simulink model "pendulum_test_model"  (R2024b)
settings: Solver=ode3  StartTime=0.0  StopTime=t(end)  RelTol=1e-3
values from neighbouring files (symbols this model uses):
  fi_dc0 = 0    [currwork.mat]    (also in pendulum_friction_coefficient_identification.m)
  g = 9.81    [currwork.mat]    (also in pendulum_friction_coefficient_identification.m)
  J_pend = 0.026668518142893    (= 0.0266685181429)    [pendulum_friction_coefficient_identification.m]
  kr = 0.026    [currwork.mat]
  kt = 0.026    [currwork.mat]
  omega_dc0 = 0    [currwork.mat]    (also in pendulum_friction_coefficient_identification.m)
  omega_pend0 = 0    [currwork.mat]    (also in pendulum_friction_coefficient_identification.m)
  R = 2.4    [currwork.mat]
  U = 0.012144    [currwork.mat]    (also in pendulum_friction_coefficient_identification.m)
  uc_dc = 0.0016    [currwork.mat]
  uc_pend = 0.00434561903982    [currwork.mat]    (also in pendulum_friction_coefficient_identification.m)
  uv_dc = 5.3017e-06    [currwork.mat]
  uv_pend = 0.000184765206116    [currwork.mat]    (also in pendulum_friction_coefficient_identification.m)
undefined symbols (not defined in the file or in its folder): J_rotor, sigbuilder_block
settings Model: Creator=Student  LastModifiedBy=Paweł Wiktor
settings SolverCC: AlgebraicLoopSolver=TrustRegion
settings DataIOCC: ReturnWorkspaceOutputs=off
settings DebuggingCC: UnconnectedInputMsg=warning  UnconnectedOutputMsg=warning  UnconnectedLineMsg=warning  ArithmeticOperatorsInVariantConditions=warning
settings ModelReferenceCC: EnableRefExpFcnMdlSchedulingChecks=on
settings SFSimCC: CustomCodeUndefinedFunction=UseInterfaceOnly
settings RTWCC: GPUComputeCapability=3.5

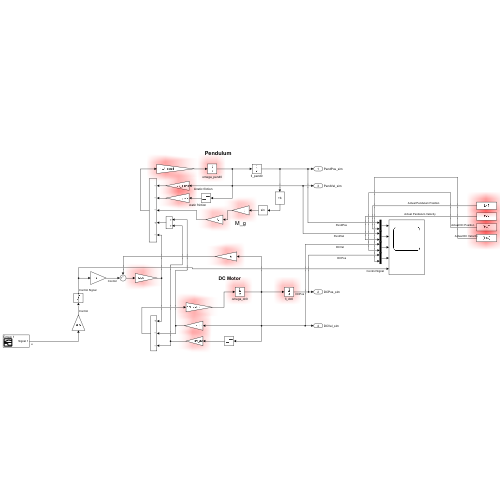
[thumbnail: Simulink's stored preview of the top-level diagram]
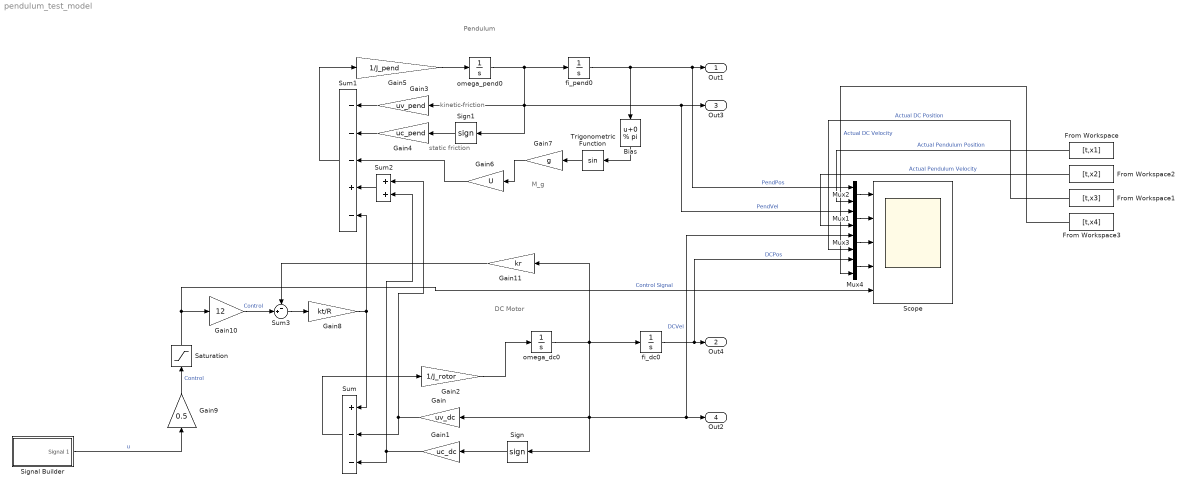
== system pendulum_test_model ==
  note: DC Motor
  note: Pendulum
  note: kinetic friction
  note: static friction
  note: M_g
  Bias : Bias  Bias=0 % pi  SaturateOnIntegerOverflow=off
  From Workspace : FromWorkspace  VariableName=[t,x1]
  From Workspace1 : FromWorkspace  VariableName=[t,x3]
  From Workspace2 : FromWorkspace  VariableName=[t,x2]
  From Workspace3 : FromWorkspace  VariableName=[t,x4]
  Gain : Gain  Gain=uv_dc
  Gain1 : Gain  Gain=uc_dc
  Gain10 : Gain  Gain=12
  Gain11 : Gain  Gain=kr
  Gain2 : Gain  Gain=1/J_rotor
  Gain3 : Gain  Gain=uv_pend
  Gain4 : Gain  Gain=uc_pend
  Gain5 : Gain  Gain=1/J_pend
  Gain6 : Gain  Gain=U
  Gain7 : Gain  Gain=g
  Gain8 : Gain  Gain=kt/R
  Gain9 : Gain  Gain=0.5
  Mux{1..4} (4 alike) : Mux  Inputs=2
  Saturation : Saturate  UpperLimit=1  LowerLimit=-1
  Scope : Scope  NumInputPorts=5
  Sign : Signum  ZeroCross=off
  Sign1 : Signum  ZeroCross=off
  Signal Builder : Subsystem  Tag=STV Subsys  LoadFcn=sigbuilder_block('load');  StartFcn=sigbuilder_block('start');  StopFcn=sigbuilder_block('stop');  ClipboardFcn=sigbuilder_block('clipboard');  mask(Sigbuilder block){tuvar=[0:10]}
      mask help: Simulink:masks:SigbuilderBlock_MD
      mask init:
      | if ~strcmp(get_param(bdroot(gcbh),'SimulationStatus'),'stopped') tuvar = sigbuilder_block('maskInit'); end
      settings: CopyFcn=sigbuilder_block('copy');  DeleteFcn=sigbuilder_block('delete');  ModelCloseFcn=sigbuilder_block('modelClose');  PreSaveFcn=sigbuilder_block('preSave');  PauseFcn=sigbuilder_block('pause');  ContinueFcn=sigbuilder_block('continue');  NameChangeFcn=sigbuilder_block('namechange');  OpenFcn=sigbuilder_block('open',[0 22.5 1440 729.75 ]);  CloseFcn=sigbuilder_block('close');
      mask Display: plot(0, 0, 100, 100,[2, 2, 32, 32, 2], [68, 8, 8, 68, 68],[32, 2], [38, 38], [32, 19, 2],[53, 60, 44], [32, 17, 17, 2],[16, 16, 31, 31]);txt = getActiveGroup(gcbh);text(2, 100, txt,'verticalAlignment', 'top');
  Sum : Sum  Inputs=+--
  Sum1 : Sum  Inputs=---+-
  Sum2 : Sum
  Sum3 : Sum  Inputs=-+|
  Trigonometric Function : Trigonometry
  fi_dc0 : Integrator  InitialCondition=fi_dc0
  fi_pend0 : Integrator  InitialCondition=0.5
  omega_dc0 : Integrator  InitialCondition=omega_dc0
  omega_pend0 : Integrator  InitialCondition=omega_pend0
  Out1 : Outport  SignalName=PendPos_sim  VectorParamsAs1DForOutWhenUnconnected=off
  Out4 : Outport  Port=2  SignalName=DCPos_sim  VectorParamsAs1DForOutWhenUnconnected=off
  Out3 : Outport  Port=3  SignalName=PendVel_sim  VectorParamsAs1DForOutWhenUnconnected=off
  Out2 : Outport  Port=4  SignalName=DCVel_sim  VectorParamsAs1DForOutWhenUnconnected=off
  wires:
  omega_dc0/1 -> Gain11/1, fi_dc0/1, Mux3/1, Out2/1, Sign/1, Gain/1  "DCVel"
  Gain2/1 -> omega_dc0/1
  Sum/1 -> Gain2/1
  Sign/1 -> Gain1/1
  Gain6/1 -> Sum1/3
  Gain7/1 -> Gain6/1
  Sum1/1 -> Gain5/1
  omega_pend0/1 -> Sign1/1, Mux1/1, Out3/1, Gain3/1, fi_pend0/1  "PendVel"
  Gain3/1 -> Sum1/1
  Trigonometric Function/1 -> Gain7/1
  fi_pend0/1 -> Mux2/1, Out1/1, Bias/1  "PendPos"
  Sign1/1 -> Gain4/1
  Gain5/1 -> omega_pend0/1
  Gain4/1 -> Sum1/2
  fi_dc0/1 -> Mux4/1, Out4/1  "DCPos"
  Gain8/1 -> Sum1/5, Sum/1
  Gain1/1 -> Sum/3, Sum2/2
  Gain/1 -> Sum/2, Sum2/1
  Sum2/1 -> Sum1/4
  Gain9/1 -> Saturation/1  "Control"
  Gain10/1 -> Sum3/2  "Control"
  Saturation/1 -> Scope/5, Gain10/1  "Control Signal"
  Sum3/1 -> Gain8/1
  Gain11/1 -> Sum3/1
  Bias/1 -> Trigonometric Function/1
  Signal Builder/1(Signal 1) -> Gain9/1  "u"
  Mux2/1 -> Scope/1
  From Workspace/1 -> Mux2/2  "Actual Pendulum Position"
  Mux1/1 -> Scope/2
  From Workspace2/1 -> Mux1/2  "Actual Pendulum Velocity"
  Mux3/1 -> Scope/3
  Mux4/1 -> Scope/4
  From Workspace1/1 -> Mux3/2  "Actual DC Position"
  From Workspace3/1 -> Mux4/2  "Actual DC Velocity"

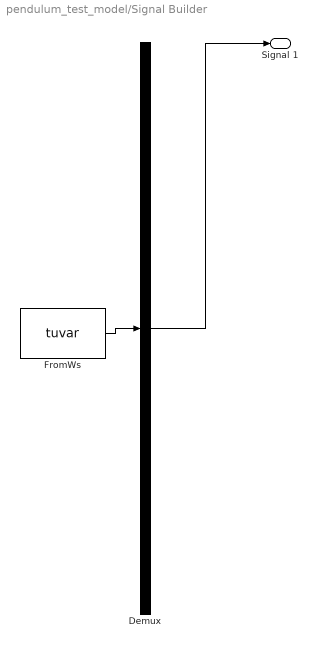
== system pendulum_test_model/Signal Builder ==
  Demux : Demux  Tag=STV Demux  Outputs=1
      settings: DisplayOption=none
  FromWs : FromWorkspace  Tag=STV FromWs  VariableName=tuvar
      SigBuilderData=|
      | common.afterFinalStr = 'Extrapolate'
      | common.sampleTime = 0
      | dataSet.timeRange = [0 10]
      | dataSet.name = 'Group 1'
      | sbobj.Groups.Name = 'Group 1'
      | sbobj.Groups.Signals.Name = 'Signal 1'
      | sbobj.Groups.Signals.XData = [0 1.98 1.98 4 4 6 6 8.32 10]
      | sbobj.Groups.Signals.YData = [0 0.17 0.51 0.37 1 1 -0.28 -0.645 0]
  Signal 1 : Outport  Tag=STV Outport  VectorParamsAs1DForOutWhenUnconnected=off
  wires:
  Demux/1 -> Signal 1/1
  FromWs/1 -> Demux/1
